simulink model "lsfirfilterdesign_tut1"  (Simulink 5.0)
settings: Solver=FixedStepDiscrete  StartTime=0.0  StopTime=inf  RelTol=1e-3
undefined symbols (not defined in the file or in its folder): get
libraries: dspddes3 x1, simulink x1, dspmtrx3 x1, dspsrcs4 x1, dspsnks4 x1
settings Model: Creator=ckamachi  LastModifiedBy=ckamachi  ExtModeTrigMode=oneshot  ExtModeArmWhenConnect=off  LimitDataPoints=off  BlockReductionOpt=off  BooleanDataType=off

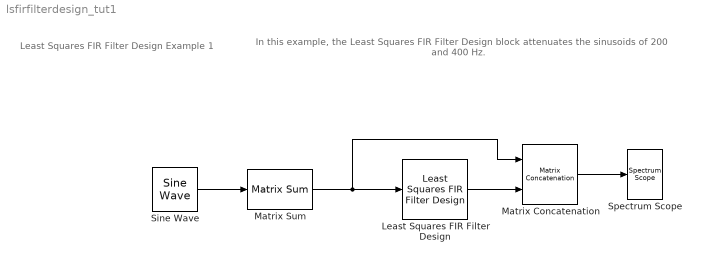
== system lsfirfilterdesign_tut1 ==
  note: Least Squares FIR Filter Design Example 1
  note: In this example, the Least Squares FIR Filter Design
      | block attenuates the sinusoids of 200 and 400 Hz.
  Least Squares FIR Filter Design : dspddes3/Least Squares FIR Filter Design  filttype=Multiband  N=16  F=[0 125 175 225 275 325 375 500]/500  A=[1 1 0 0 1 1 0 0]  W=[1 1 1 1]
  Matrix Concatenation : simulink/Math Operations/Matrix Concatenation  numInports=2  catMethod=Horizontal
  Matrix Sum : dspmtrx3/Matrix Sum  Dim=Rows
  Sine Wave : dspsrcs4/Sine Wave  Amplitude=10  Frequency=[100 200 300 400]  Phase=0  SampleMode=Discrete  OutComplex=Real  CompMethod=Trigonometric fcn  TableSize=Speed  SampleTime=0.001  SamplesPerFrame=128  dataType=double  wordLen=16  udDataType=sfix(16)  fracBitsMode=Best precision  numFracBits=14  ResetState=Restart at time zero
  Spectrum Scope : dspsnks4/Spectrum Scope  ScopeProperties=on  Domain=Frequency  HorizSpan=1  UseBuffer=off  BufferSize=128  Overlap=64  inpFftLenInherit=off  FFTlength=128  numAvg=2  DisplayProperties=off  AxisGrid=on  Memory=off  FrameNumber=on  AxisLegend=off  AxisZoom=off  OpenScopeAtSimStart=on  OpenScopeImmediately=off  FigPos=get(0,'defaultfigureposition')  AxisProperties=off  XUnits=Hertz  XRange=[0...Fs/2]  InheritXIncr=on  XIncr=1.0  XLabel=Samples  YUnits=dB  YLabel=Magnitude, dB  LineProperties=off  LineColors=[0 0 1]
      settings: YMin=-88.6943683511669  YMax=34.6872027325711
  wires:
  Sine Wave/1 -> Matrix Sum/1
  Matrix Sum/1 -> Least Squares FIR Filter Design/1, Matrix Concatenation/1
  Least Squares FIR Filter Design/1 -> Matrix Concatenation/2
  Matrix Concatenation/1 -> Spectrum Scope/1
